simulink model "ejercicio1"  (R2020a)
settings: Solver=VariableStepAuto  StartTime=0.0  StopTime=4500  RelTol=1e-3
settings Model: Creator=joaqu  LastModifiedBy=joaqu

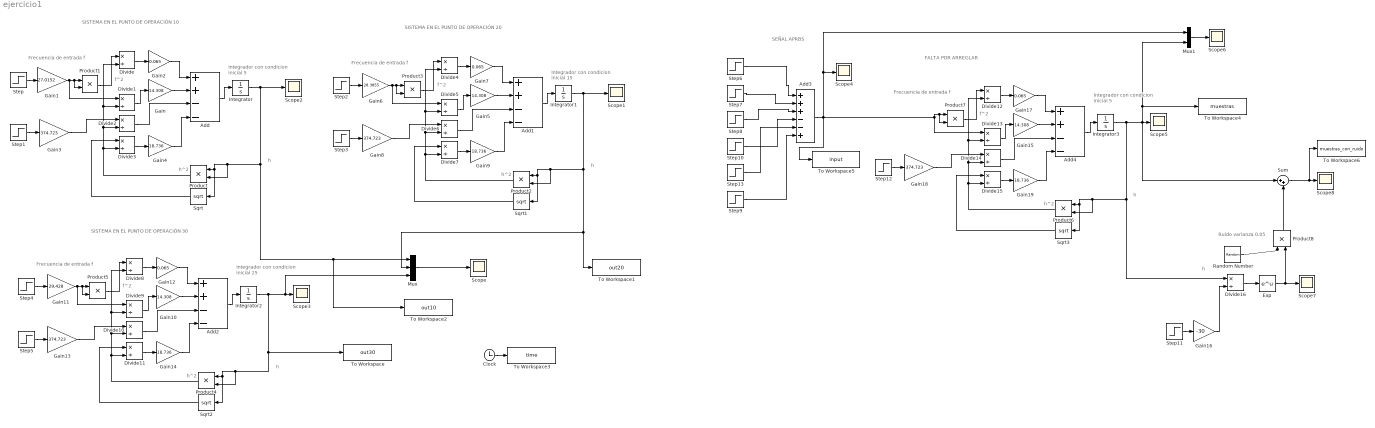
== system ejercicio1 ==
  note: h^2
  note: h
  note: Integrador con
      |  condicion inicial 5
  note: SISTEMA EN EL PUNTO DE OPERACIÓN 10
  note: Frecuencia de entrada
      | 		f
  note: f^2
  note: f^2
  note: SISTEMA EN EL PUNTO DE OPERACIÓN 20
  note: Frecuencia de entrada
      | 		f
  note: h^2
  note: h
  note: Integrador con
      |  condicion inicial 15
  note: h
  note: Frecuencia de entrada
      | 		f
  note: SISTEMA EN EL PUNTO DE OPERACIÓN 30
  note: h^2
  note: f^2
  note: Integrador con
      |  condicion inicial 25
  note: SEÑAL APRBS
  note: Frecuencia de entrada
      | 		f
  note: f^2
  note: h^2
  note: h
  note: Integrador con
      |  condicion inicial 5
  note: FALTA POR ARREGLAR
  note: h
  note: Ruido varianza
      | 0.05
  Add{,1..2,4} (4 alike) : Sum  Inputs=++--
  Add3 : Sum  Inputs=+++--+
  Clock : Clock
  Divide{,1..16} (17 alike) : Product  Inputs=*/
  Exp : Math  SaturateOnIntegerOverflow=on
  Gain{,5,10,15} (4 alike) : Gain  Gain=14.308
  Gain1 : Gain  Gain=27.0152
  Gain11 : Gain  Gain=29.428
  Gain{2,7,12,17} (4 alike) : Gain  Gain=0.065
  Gain{3,8,13,18} (4 alike) : Gain  Gain=374.723
  Gain{4,9,14,19} (4 alike) : Gain  Gain=18.736
  Gain16 : Gain  Gain=-30
  Gain6 : Gain  Gain=28.3855
  Integrator : Integrator  InitialCondition=5
  Integrator1 : Integrator  InitialCondition=15
  Integrator2 : Integrator  InitialCondition=25
  Integrator3 : Integrator  InitialCondition=5
  Mux : Mux  Inputs=3
  Mux1 : Mux  Inputs=2
  Product{,1..8} (9 alike) : Product
  Random Number : RandomNumber  Variance=0.05  SampleTime=5
  Scope{,1..8} (9 alike) : Scope
  Sqrt{,1..3} (4 alike) : Sqrt  SaturateOnIntegerOverflow=on
  Step{,1..5,11..12} (8 alike) : Step  Time=0  SampleTime=0
  Step10 : Step  Time=2151  After=1.043  SampleTime=0
  Step13 : Step  Time=2751  After=1.3705  SampleTime=0
  Step6 : Step  Time=126  Before=27.015  After=0  SampleTime=0
  Step7 : Step  Time=126  After=28.386  SampleTime=0
  Step8 : Step  Time=726  After=1.043  SampleTime=0
  Step9 : Step  Time=2877  After=2.4129  SampleTime=0
  Sum : Sum  Inputs=|++
  To Workspace : ToWorkspace  VariableName=out30  SampleTime=-1
      settings: Save2DSignal=2-D array (concatenate along first dimension)
  To Workspace1 : ToWorkspace  VariableName=out20  SampleTime=-1
      settings: Save2DSignal=2-D array (concatenate along first dimension)
  To Workspace2 : ToWorkspace  VariableName=out10  SampleTime=-1
      settings: Save2DSignal=2-D array (concatenate along first dimension)
  To Workspace3 : ToWorkspace  VariableName=time  SaveFormat=Timeseries  SampleTime=-1
  To Workspace4 : ToWorkspace  VariableName=muestras  SampleTime=-1
      settings: Save2DSignal=2-D array (concatenate along first dimension)
  To Workspace5 : ToWorkspace  VariableName=input  SampleTime=-1
      settings: Save2DSignal=2-D array (concatenate along first dimension)
  To Workspace6 : ToWorkspace  VariableName=muestras_con_ruido  SampleTime=-1
      settings: Save2DSignal=2-D array (concatenate along first dimension)
  wires:
  Step/1 -> Gain1/1
  Add/1 -> Integrator/1
  Integrator/1 -> Mux/1, To Workspace2/1, Product/2, Product/1, Sqrt/1, Scope2/1
  Gain1/1 -> Divide1/1, Product1/2, Product1/1
  Product1/1 -> Divide/1
  Product/1 -> Divide3/2, Divide2/2, Divide1/2, Divide/2
  Divide/1 -> Gain2/1
  Gain2/1 -> Add/1
  Divide2/1 -> Add/3
  Sqrt/1 -> Divide3/1
  Step1/1 -> Gain3/1
  Gain3/1 -> Divide2/1
  Gain/1 -> Add/2
  Divide1/1 -> Gain/1
  Divide3/1 -> Gain4/1
  Gain4/1 -> Add/4
  Divide5/1 -> Gain5/1
  Divide7/1 -> Gain9/1
  Divide4/1 -> Gain7/1
  Step3/1 -> Gain8/1
  Gain8/1 -> Divide6/1
  Product3/1 -> Divide4/1
  Gain5/1 -> Add1/2
  Sqrt1/1 -> Divide7/1
  Gain9/1 -> Add1/4
  Step2/1 -> Gain6/1
  Product2/1 -> Divide7/2, Divide6/2, Divide5/2, Divide4/2
  Gain6/1 -> Divide5/1, Product3/2, Product3/1
  Divide6/1 -> Add1/3
  Add1/1 -> Integrator1/1
  Gain7/1 -> Add1/1
  Divide10/1 -> Add2/3
  Add2/1 -> Integrator2/1
  Divide9/1 -> Gain10/1
  Step4/1 -> Gain11/1
  Product4/1 -> Divide11/2, Divide10/2, Divide9/2, Divide8/2
  Integrator2/1 -> Mux/3, Scope3/1, Product4/2, Product4/1, Sqrt2/1, To Workspace/1
  Product5/1 -> Divide8/1
  Gain14/1 -> Add2/4
  Gain10/1 -> Add2/2
  Sqrt2/1 -> Divide11/1
  Divide8/1 -> Gain12/1
  Divide11/1 -> Gain14/1
  Gain13/1 -> Divide10/1
  Gain11/1 -> Divide9/1, Product5/2, Product5/1
  Step5/1 -> Gain13/1
  Gain12/1 -> Add2/1
  Mux/1 -> Scope/1
  Integrator1/1 -> Scope1/1, Mux/2, To Workspace1/1, Product2/2, Product2/1, Sqrt1/1
  Clock/1 -> To Workspace3/1
  Step7/1 -> Add3/2
  Step6/1 -> Add3/1
  Step8/1 -> Add3/3
  Step10/1 -> Add3/4
  Step13/1 -> Add3/5
  Step9/1 -> Add3/6
  Sqrt3/1 -> Divide15/1
  Divide15/1 -> Gain19/1
  Add3/1 -> To Workspace5/1, Product7/2, Product7/1, Divide13/1, Mux1/1, Scope4/1
  Add4/1 -> Integrator3/1
  Gain19/1 -> Add4/4
  Gain17/1 -> Add4/1
  Gain15/1 -> Add4/2
  Gain18/1 -> Divide14/1
  Step12/1 -> Gain18/1
  Divide13/1 -> Gain15/1
  Product6/1 -> Divide15/2, Divide14/2, Divide13/2, Divide12/2
  Product7/1 -> Divide12/1
  Divide12/1 -> Gain17/1
  Divide14/1 -> Add4/3
  Mux1/1 -> Scope6/1
  Integrator3/1 -> Divide16/1, Product6/2, Product6/1, Sqrt3/1, Mux1/2, To Workspace4/1, Scope5/1, Sum/1
  Exp/1 -> Scope7/1, Product8/2
  Step11/1 -> Gain16/1
  Product8/1 -> Sum/2
  Gain16/1 -> Divide16/2
  Random Number/1 -> Product8/1
  Divide16/1 -> Exp/1
  Sum/1 -> To Workspace6/1, Scope8/1
